simulink model "Ex32"  (R2021b)
settings: Solver=VariableStepAuto  StartTime=0.0  StopTime=10  RelTol=1e-3
settings Model: Creator=abdul  LastModifiedBy=abdul

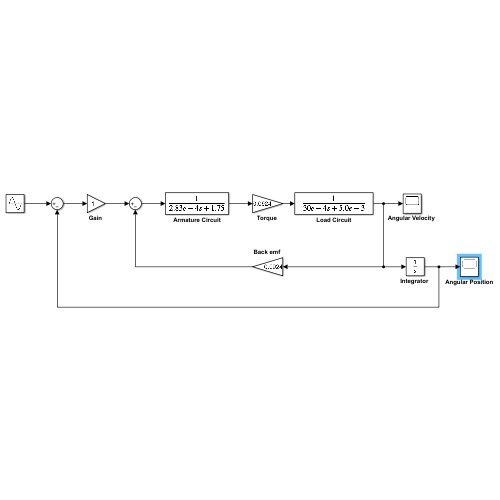
[thumbnail: Simulink's stored preview of the top-level diagram]
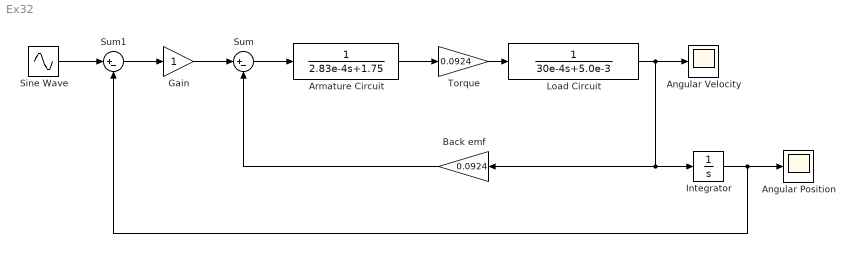
== system Ex32 ==
  Angular Position : Scope
  "Angular Velocity " : Scope
  Armature Circuit : TransferFcn  Denominator=[2.83e-4 1.75]
  "Back emf " : Gain  Gain=0.0924
  "Gain " : Gain
  "Integrator " : Integrator
  Load Circuit : TransferFcn  Denominator=[30e-4 5.0e-3]
  Sine Wave : Sin  SampleTime=0
  Sum : Sum  Inputs=|+-
  Sum1 : Sum  Inputs=|+-
  "Torque " : Gain  Gain=0.0924
  wires:
  Sum/1 -> Armature Circuit/1
  Armature Circuit/1 -> "Torque "/1
  "Torque "/1 -> Load Circuit/1
  "Back emf "/1 -> Sum/2
  Load Circuit/1 -> "Angular Velocity "/1, "Integrator "/1, "Back emf "/1
  Sum1/1 -> "Gain "/1
  "Gain "/1 -> Sum/1
  Sine Wave/1 -> Sum1/1
  "Integrator "/1 -> Angular Position/1, Sum1/2
